simulink model "decoupled_dynamics"  (R2021a)
settings: Solver=ode45  StartTime=0.0  StopTime=10.0  RelTol=1e-3
values from neighbouring files (symbols this model uses):
  A_dT_PD = double(A(3:4,3:4))    [Linearize_Fast.m]
  A_dt_PN = double(A(1:2,1:2))    [Linearize_Fast.m]
  A_dt_psi = double(A(11:12,11:12))    [Linearize_Fast.m]
  A_dt_u = double(A(8:10,8:10))    [Linearize_Fast.m]
  A_dt_v = double(A(5:7,5:7))    [Linearize_Fast.m]
  B_dT_PD = double(B(3:4,1))    [Linearize_Fast.m]
  B_dt_PN = double([A(1,8) A(1,11);A(2,8) A(2,11)])    [Linearize_Fast.m]
  B_dt_psi = double(B(11:12,4))    [Linearize_Fast.m]
  B_dt_u = double(B(8:10, 3))    [Linearize_Fast.m]
  B_dt_v = double(B(5:7, 2))    [Linearize_Fast.m]
  ic_u = [0.6522;0;0;0]    [Linearize_Fast.m]
  x0 = [0; 0; -1; sin(-.2119); 0; 0; 0; cos(.2119); -.2119; 0; 0; 0;]    [Linearize_Fast.m]
  xhover = [0; 0; -1; 0; 0; 0; 0; 0; 0; 0; 0; 0;]    [Linearize_Fast.m]
undefined symbols (not defined in the file or in its folder): K_PD, K_psi, K_u, K_v
settings Model: Creator=Willi  LastModifiedBy=jtc12

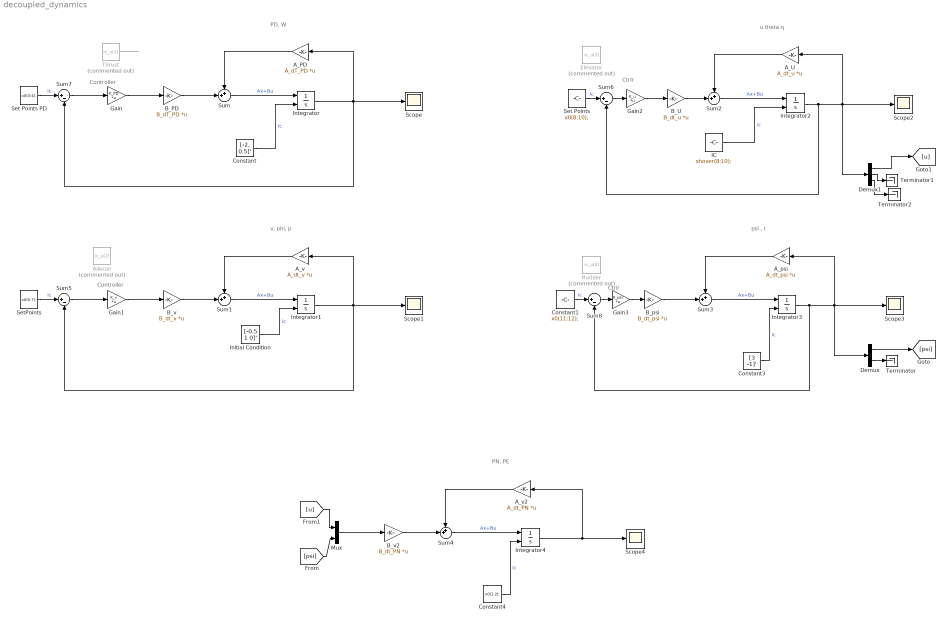
== system decoupled_dynamics ==
  note: Ctrlr
  note: Controller
  note: Ctrlr
  note: Controller
  note: PD, W
  note: v, phi, p
  note: u theta q
  note: psi , r
  note: PN, PE
  A_PD : Gain  Gain=A_dT_PD  Multiplication=Matrix(K*u)
  A_U : Gain  Gain=A_dt_u  Multiplication=Matrix(K*u)
  A_psi : Gain  Gain=A_dt_psi  Multiplication=Matrix(K*u)
  A_v : Gain  Gain=A_dt_v  Multiplication=Matrix(K*u)
  A_v2 : Gain  Gain=A_dt_PN  Multiplication=Matrix(K*u)
  Aileron : Constant  Commented=on  Value=ic_u(2)
  B_PD : Gain  Gain=B_dT_PD  Multiplication=Matrix(K*u)
  B_U : Gain  Gain=B_dt_u  Multiplication=Matrix(K*u)
  B_psi : Gain  Gain=B_dt_psi  Multiplication=Matrix(K*u)
  B_v : Gain  Gain=B_dt_v  Multiplication=Matrix(K*u)
  B_v2 : Gain  Gain=B_dt_PN  Multiplication=Matrix(K*u)
  Constant : Constant  Value=[-2, 0.5]'
  Constant1 : Constant  Value=x0(11:12);
  Constant3 : Constant  Value=[3 -1]'
  Constant4 : Constant  Value=x0(1:2);
  Demux : Demux  Outputs=2
  Demux1 : Demux  Outputs=3
  Elevator : Constant  Commented=on  Value=ic_u(3)
  Gain : Gain  Gain=K_PD  Multiplication=Matrix(K*u)
  Gain1 : Gain  Gain=K_v  Multiplication=Matrix(K*u)
  Gain2 : Gain  Gain=K_u  Multiplication=Matrix(K*u)
  Gain3 : Gain  Gain=K_psi  Multiplication=Matrix(K*u)
  IC : Constant  Value=xhover(8:10);
  Initial Condition : Constant  Value=[-0.5 1 0]'
  Integrator{,1..4} (5 alike) : Integrator  InitialConditionSource=external
  Mux : Mux  Inputs=2
  Rudder : Constant  Commented=on  Value=ic_u(4)
  Scope{,1..4} (5 alike) : Scope
  Set Points : Constant  Value=x0(8:10);
  Set Points PD : Constant  Value=x0(3:4);
  SetPoints : Constant  Value=x0(5:7);
  Sum{,1..4} (5 alike) : Sum  Inputs=++|
  Sum{5..8} (4 alike) : Sum  Inputs=|+-
  Terminator : Terminator
  Terminator1 : Terminator
  Terminator2 : Terminator
  Thrust : Constant  Commented=on  Value=ic_u(1)
  wires:
  Integrator/1 -> Scope/1, Sum7/2, A_PD/1
  Constant/1 -> Integrator/2  "ic"
  A_PD/1 -> Sum/1
  B_PD/1 -> Sum/2
  Sum/1 -> Integrator/1  "Ax+Bu"
  Thrust/1 -> ?
  Sum1/1 -> Integrator1/1  "Ax+Bu"
  B_v/1 -> Sum1/2
  A_v/1 -> Sum1/1
  Initial Condition/1 -> Integrator1/2  "ic"
  Integrator1/1 -> Scope1/1, Sum5/2, A_v/1
  Integrator3/1 -> Scope3/1, Demux/1, A_psi/1, Sum8/2
  Constant3/1 -> Integrator3/2  "ic"
  A_psi/1 -> Sum3/1
  B_psi/1 -> Sum3/2
  Sum3/1 -> Integrator3/1  "Ax+Bu"
  Sum2/1 -> Integrator2/1  "Ax+Bu"
  B_U/1 -> Sum2/2
  A_U/1 -> Sum2/1
  IC/1 -> Integrator2/2  "ic"
  Mux/1 -> B_v2/1
  Sum4/1 -> Integrator4/1  "Ax+Bu"
  B_v2/1 -> Sum4/2
  A_v2/1 -> Sum4/1
  Constant4/1 -> Integrator4/2  "ic"
  Integrator4/1 -> A_v2/1, Scope4/1
  Demux/2 -> Terminator/1
  Demux/1 -> [psi]
  [psi] -> Mux/2
  Demux1/1 -> [u]
  Demux1/2 -> Terminator1/1
  Integrator2/1 -> Demux1/1, Scope2/1, A_U/1, Sum6/2
  [u] -> Mux/1
  Demux1/3 -> Terminator2/1
  SetPoints/1 -> Sum5/1  "ic"
  Sum5/1 -> Gain1/1
  Gain1/1 -> B_v/1
  Set Points/1 -> Sum6/1  "ic"
  Sum6/1 -> Gain2/1
  Gain2/1 -> B_U/1
  Gain/1 -> B_PD/1
  Sum7/1 -> Gain/1
  Set Points PD/1 -> Sum7/1  "ic"
  Gain3/1 -> B_psi/1
  Constant1/1 -> Sum8/1  "ic"
  Sum8/1 -> Gain3/1
